simulink model "gesteuerte_Kreisfahrt"  (R2023a)
settings: Solver=VariableStepAuto  StartTime=0.0  StopTime=10.0  RelTol=1e-3
values from neighbouring files (symbols this model uses):
  v = 60 / 3.6    (= 16.6666666667)    [geregelte_kreisfahrt.m]    (also in gesteuerte_kreisfahrt.m)
undefined symbols (not defined in the file or in its folder): C, D, iS, J, Lh, Lv, m
libraries: simulink x2
settings Model: Creator=victoriastrobel  LastModifiedBy=nova

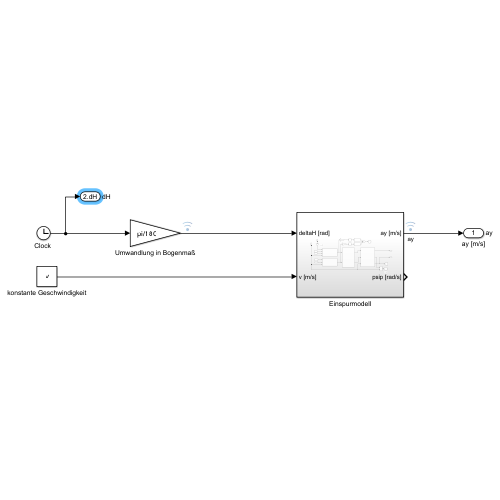
[thumbnail: Simulink's stored preview of the top-level diagram]
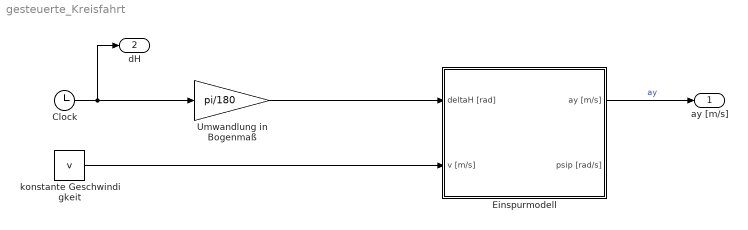
== system gesteuerte_Kreisfahrt ==
  "Clock " : Clock
  Einspurmodell : Subsystem
  Umwandlung in Bogenmaß : Gain  Gain=pi/180
  konstante Geschwindigkeit : Constant  Value=v
  ay [m/s] : Outport  SignalName=ay  SampleTime=0.01
  dH : Outport  Port=2  SignalName=dH  SampleTime=0.01
  wires:
  Einspurmodell/1(ay [m/s]) -> ay [m/s]/1  "ay"
  konstante Geschwindigkeit/1 -> Einspurmodell/2(v [m/s])
  "Clock "/1 -> Umwandlung in Bogenmaß/1, dH/1
  Umwandlung in Bogenmaß/1 -> Einspurmodell/1(deltaH [rad])

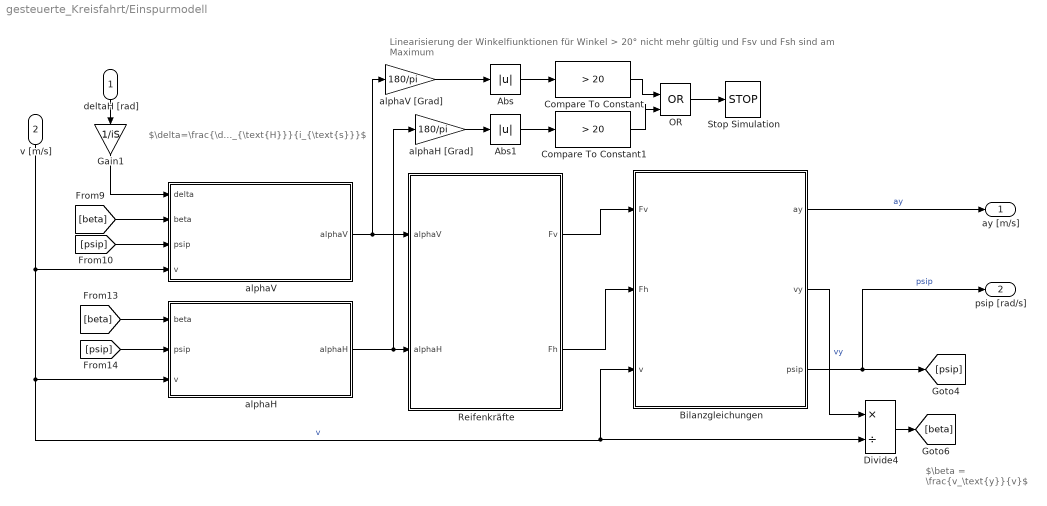
== system gesteuerte_Kreisfahrt/Einspurmodell ==
  note: Linearisierung der Winkelfiunktionen für Winkel > 20° nicht mehr gültig und Fsv und Fsh sind am Maximum
  note: $\beta = \frac{v_\text{y}}{v}$
  note: $\delta=\frac{\delta_{\text{H}}}{i_{\text{s}}}$
  deltaH [rad] : Inport
  v [m/s] : Inport  Port=2
  Abs : Abs  SaturateOnIntegerOverflow=off
  Abs1 : Abs  SaturateOnIntegerOverflow=off
  Bilanzgleichungen : Subsystem
  Compare To Constant : simulink/Logic and Bit Operations/Compare To Constant  relop=>  const=20  OutDataTypeStr=boolean
  Compare To Constant1 : simulink/Logic and Bit Operations/Compare To Constant  relop=>  const=20  OutDataTypeStr=boolean
  Divide4 : Product  Inputs=*/
  Gain1 : Gain  Gain=1/iS
  OR : Logic  Operator=OR  IconShape=distinctive  AllPortsSameDT=off  OutDataTypeStr=boolean
  Reifenkräfte : Subsystem
  Stop Simulation : Stop
  alphaH : Subsystem
  alphaH [Grad] : Gain  Gain=180/pi
  alphaV : Subsystem
  alphaV [Grad] : Gain  Gain=180/pi
  ay [m/s] : Outport
  psip [rad/s] : Outport  Port=2
  wires:
  v [m/s]/1 -> Bilanzgleichungen/3(v), Divide4/2, alphaH/3(v), alphaV/4(v)  "v"
  Bilanzgleichungen/2(vy) -> Divide4/1  "vy"
  Divide4/1 -> [beta]
  [beta] -> alphaH/1(beta)
  [psip] -> alphaH/2(psip)
  alphaH/1(alphaH) -> alphaH [Grad]/1, Reifenkräfte/2(alphaH)
  deltaH [rad]/1 -> Gain1/1
  [beta] -> alphaV/2(beta)
  [psip] -> alphaV/3(psip)
  alphaV/1(alphaV) -> alphaV [Grad]/1, Reifenkräfte/1(alphaV)
  Bilanzgleichungen/1(ay) -> ay [m/s]/1  "ay"
  Reifenkräfte/1(Fv) -> Bilanzgleichungen/1(Fv)
  Reifenkräfte/2(Fh) -> Bilanzgleichungen/2(Fh)
  Bilanzgleichungen/3(psip) -> psip [rad/s]/1, [psip]  "psip"
  Compare To Constant/1 -> OR/1
  Compare To Constant1/1 -> OR/2
  OR/1 -> Stop Simulation/1
  Gain1/1 -> alphaV/1(delta)
  Abs/1 -> Compare To Constant/1
  alphaH [Grad]/1 -> Abs1/1
  Abs1/1 -> Compare To Constant1/1
  alphaV [Grad]/1 -> Abs/1

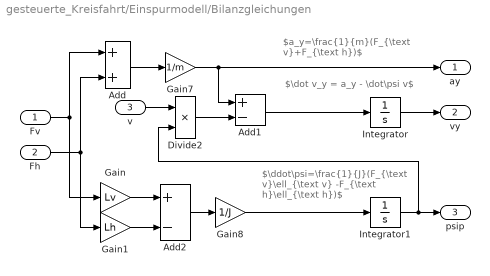
== system gesteuerte_Kreisfahrt/Einspurmodell/Bilanzgleichungen ==
  note: $\ddot\psi=\frac{1}{J}(F_{\text v}\ell_{\text v} -F_{\text h}\ell_{\text h})$
  note: $\dot v_y = a_y - \dot\psi v$
  note: $a_y=\frac{1}{m}(F_{\text v}+F_{\text h})$
  Fv : Inport
  Fh : Inport  Port=2
  v : Inport  Port=3
  Add : Sum
  Add1 : Sum  Inputs=+-
  Add2 : Sum  Inputs=+-
  Divide2 : Product  Inputs=**
  Gain : Gain  Gain=Lv
  Gain1 : Gain  Gain=Lh
  Gain7 : Gain  Gain=1/m
  Gain8 : Gain  Gain=1/J
  Integrator : Integrator
  Integrator1 : Integrator
  ay : Outport
  vy : Outport  Port=2
  psip : Outport  Port=3
  wires:
  Fh/1 -> Add/2, Gain1/1
  Integrator/1 -> vy/1
  Add2/1 -> Gain8/1
  v/1 -> Divide2/1
  Gain/1 -> Add2/1
  Divide2/1 -> Add1/2
  Gain7/1 -> ay/1, Add1/1
  Gain8/1 -> Integrator1/1
  Fv/1 -> Gain/1, Add/1
  Gain1/1 -> Add2/2
  Integrator1/1 -> Divide2/2, psip/1
  Add/1 -> Gain7/1
  Add1/1 -> Integrator/1

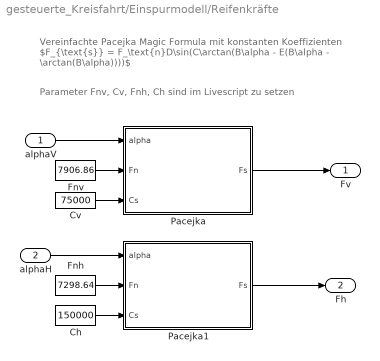
== system gesteuerte_Kreisfahrt/Einspurmodell/Reifenkräfte ==
  note: Parameter Fnv, Cv, Fnh, Ch sind im Livescript zu setzen
  note: Vereinfachte Pacejka Magic Formula mit konstanten Koeffizienten
      | $F_{\text{s}} = F_\text{n}D\sin(C\arctan(B\alpha - E(B\alpha - \arctan(B\alpha))))$
  alphaV : Inport
  alphaH : Inport  Port=2
  Ch : Constant  Value=150000
  Cv : Constant  Value=75000
  Fnh : Constant  Value=7298.64
  Fnv : Constant  Value=7906.86
  Pacejka : MATLAB Function  TreatAsAtomicUnit=on
  Pacejka1 : MATLAB Function  TreatAsAtomicUnit=on
  Fv : Outport
  Fh : Outport  Port=2
  wires:
  alphaV/1 -> Pacejka/1(alpha)
  alphaH/1 -> Pacejka1/1(alpha)
  Fnv/1 -> Pacejka/2(Fn)
  Pacejka/1(Fs) -> Fv/1
  Pacejka1/1(Fs) -> Fh/1
  Cv/1 -> Pacejka/3(Cs)
  Fnh/1 -> Pacejka1/2(Fn)
  Ch/1 -> Pacejka1/3(Cs)

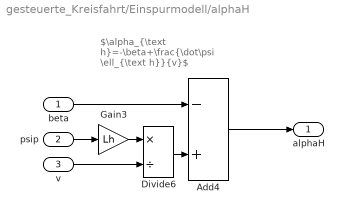
== system gesteuerte_Kreisfahrt/Einspurmodell/alphaH ==
  note: $\alpha_{\text h}=-\beta+\frac{\dot\psi \ell_{\text h}}{v}$
  beta : Inport
  psip : Inport  Port=2
  v : Inport  Port=3
  Add4 : Sum  Inputs=-+
  Divide6 : Product  Inputs=*/
  Gain3 : Gain  Gain=Lh
  alphaH : Outport
  wires:
  v/1 -> Divide6/2
  psip/1 -> Gain3/1
  Add4/1 -> alphaH/1
  beta/1 -> Add4/1
  Gain3/1 -> Divide6/1
  Divide6/1 -> Add4/2

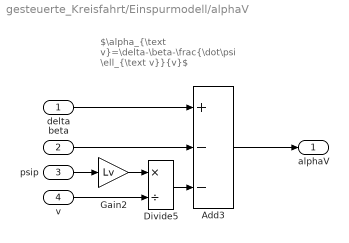
== system gesteuerte_Kreisfahrt/Einspurmodell/alphaV ==
  note: $\alpha_{\text v}=\delta-\beta-\frac{\dot\psi \ell_{\text v}}{v}$
  delta : Inport
  beta : Inport  Port=2
  psip : Inport  Port=3
  v : Inport  Port=4
  Add3 : Sum  Inputs=+--
  Divide5 : Product  Inputs=*/
  Gain2 : Gain  Gain=Lv
  alphaV : Outport
  wires:
  Add3/1 -> alphaV/1
  v/1 -> Divide5/2
  Gain2/1 -> Divide5/1
  delta/1 -> Add3/1
  beta/1 -> Add3/2
  psip/1 -> Gain2/1
  Divide5/1 -> Add3/3

== matlab function gesteuerte_Kreisfahrt/Einspurmodell/Reifenkräfte/Pacejka1 ==
  settings: updateMethod=DISCRETE
  data: alpha input; Fs output; Fn input; Cs input; C parameter; D parameter; E parameter
function Fs  = Pacejka(alpha, Fn, Cs, C, D, E)
% alpha: Schräglaufwinkel in rad
% Fn: Normalkraft in N
% Cs: Schräglaufsteifigkeit in N/rad
% C, D, E: Pacejka-Paramter
% https://de.mathworks.com/help/sdl/ref/tireroadinteractionmagicformula.html
% https://www.edy.es/dev/docs/pacejka-94-parameters-explained-a-comprehensive-guide/
B = Cs/Fn/C/D;
Fs = Fn*D*sin(C*atan(B*alpha - E*(B*alpha - atan(B*alpha))));

== matlab function gesteuerte_Kreisfahrt/Einspurmodell/Reifenkräfte/Pacejka ==
  settings: updateMethod=DISCRETE
  data: alpha input; Fs output; Fn input; Cs input; C parameter; D parameter; E parameter
function Fs  = Pacejka(alpha, Fn, Cs, C, D, E)
% alpha: Schräglaufwinkel in rad
% Fn: Normalkraft in N
% Cs: Schräglaufsteifigkeit in N/rad
% C, D, E: Pacejka-Paramter
% https://de.mathworks.com/help/sdl/ref/tireroadinteractionmagicformula.html
% https://www.edy.es/dev/docs/pacejka-94-parameters-explained-a-comprehensive-guide/
B = Cs/Fn/C/D;
Fs = Fn*D*sin(C*atan(B*alpha - E*(B*alpha - atan(B*alpha))));
